simulink model "Automatisierung_subsystem_test"  (R2016b)
settings: Solver=FixedStepAuto  StartTime=0.0  StopTime=80.0  FixedStep=0.001  RelTol=1e-3
model workspace (MAT data in the model file):
  a = Simulink.Parameter
  a.DataType = 'auto'
  a.Dimensions = [0 0]
  b = Simulink.Parameter
  b.DataType = 'auto'
  b.Dimensions = [0 0]
settings Model: Creator=Fritz  LastModifiedBy=Fritz

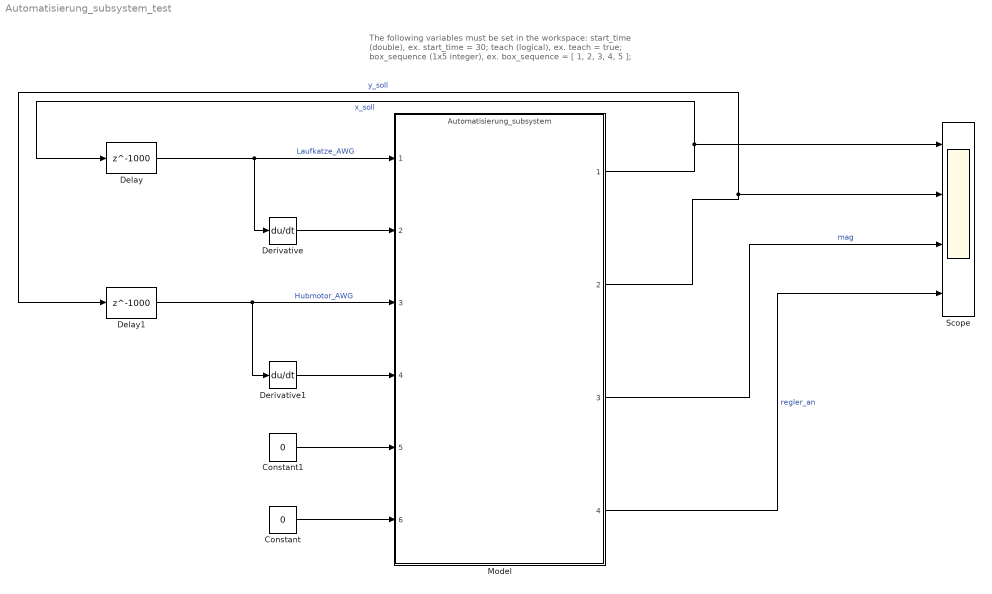
== system Automatisierung_subsystem_test ==
  note: The following variables must be set in the workspace:
      | start_time (double), ex. start_time = 30;
      | teach (logical), ex. teach = true;
      | box_sequence (1x5 integer), ex. box_sequence = [ 1, 2, 3, 4, 5 ];
  Constant : Constant  Value=0  OutDataTypeStr=double
  Constant1 : Constant  Value=0  OutDataTypeStr=double
  Delay : Delay  DelayLength=1000
  Delay1 : Delay  DelayLength=1000
  Derivative : Derivative
  Derivative1 : Derivative
  Model : ModelReference  ModelNameDialog=Automatisierung_subsystem.slx  SimulationMode=Normal  ModelReferenceVersion=1.100
  Scope : Scope  NumInputPorts=4
  wires:
  Model/1 -> Scope/1, Delay/1  "x_soll"
  Model/2 -> Scope/2, Delay1/1  "y_soll"
  Model/3 -> Scope/3  "mag"
  Model/4 -> Scope/4  "regler_an"
  Delay/1 -> Model/1, Derivative/1  "Laufkatze_AWG"
  Delay1/1 -> Model/3, Derivative1/1  "Hubmotor_AWG"
  Constant/1 -> Model/6
  Constant1/1 -> Model/5
  Derivative1/1 -> Model/4
  Derivative/1 -> Model/2
